simulink model "Helicopter_2_DOF"  (R2013b)
settings: Solver=ode45  StartTime=0.0  StopTime=10.0  RelTol=1e-3
InitFcn:
  | load('Matrizes.mat');
  | load('Ganhos.mat');
values from neighbouring files (symbols this model uses):
  A = 10^-4    (= 0.0001)    [CustoHinf.m]    (also in Linearizacao.m = double(subs(A)); Matrizes.mat = [0 0 0 0 1 -8.77274061048 0 0 0 0 0 0 ... (16 elements, 4x4))
  B = double(subs(B))    [Linearizacao.m]    (also in Matrizes.mat = [0  0; 2.23704885567  0.0745682951891; 0  0; 0.253496952258 )
  C = double(subs(C))    [Linearizacao.m]    (also in Matrizes.mat = [1  0  0  0; 0  0  1  0])
  D = double(subs(D))    [Linearizacao.m]    (also in Matrizes.mat = [0  0; 0  0])
  k1 = x(1)    [Custo.m]    (also in CustoHinf.m; Ganhos.mat = 728.989958125; Main.m)
  k2 = x(2)    [Custo.m]    (also in CustoHinf.m; Ganhos.mat = -330.932991599; Main.m)
  k3 = x(3)    [Custo.m]    (also in CustoHinf.m; Ganhos.mat = 1028.64172703; Main.m)
  k4 = x(4)    [Custo.m]    (also in CustoHinf.m; Ganhos.mat = -351.190963552; Main.m)
settings Model: Creator=Eduardo  LastModifiedBy=Eduardo

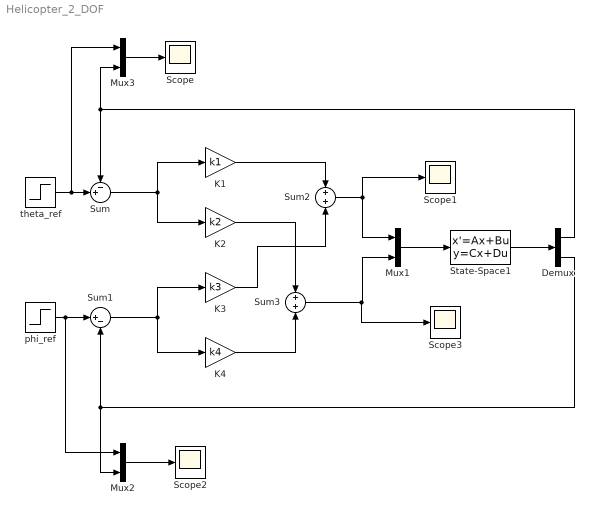
== system Helicopter_2_DOF ==
  Demux : Demux  Outputs=2
  K1 : Gain  Gain=k1
  "K2 " : Gain  Gain=k2
  K3 : Gain  Gain=k3
  "K4 " : Gain  Gain=k4
  Mux1 : Mux  Inputs=2
  Mux2 : Mux  Inputs=2
  Mux3 : Mux  Inputs=2
  Scope{,1..3} (4 alike) : Scope
      Scope2 settings: SaveName=ScopeData2
      Scope3 settings: SaveName=ScopeData3
  State-Space1 : StateSpace  A=A  B=B  C=C  D=D  X0=0
  Sum : Sum  Inputs=-+|
  Sum1 : Sum  Inputs=|+-
  Sum2 : Sum  Inputs=+|+
  Sum3 : Sum  Inputs=+|+
  phi_ref : Step  Time=5  SampleTime=0
  theta_ref : Step  SampleTime=0
  wires:
  theta_ref/1 -> Mux3/1, Sum/2
  State-Space1/1 -> Demux/1
  Demux/1 -> Mux3/2, Sum/1
  Demux/2 -> Mux2/2, Sum1/2
  phi_ref/1 -> Mux2/1, Sum1/1
  Mux1/1 -> State-Space1/1
  Sum/1 -> K1/1, "K2 "/1
  Sum1/1 -> K3/1, "K4 "/1
  K1/1 -> Sum2/1
  K3/1 -> Sum2/2
  "K2 "/1 -> Sum3/1
  "K4 "/1 -> Sum3/2
  Mux3/1 -> Scope/1
  Mux2/1 -> Scope2/1
  Sum2/1 -> Mux1/1, Scope1/1
  Sum3/1 -> Scope3/1, Mux1/2
